simulink library "MonoizerLib"  (R2022b)
settings: Solver=VariableStepAuto  StartTime=0.0  StopTime=10.0  RelTol=1e-3
libraries: TuneVar x2, dspindex x2, HandyTextFile x1, matrix_library x1
settings Model: Creator=jb1046154  LastModifiedBy=sa1045272
settings SolverCC: AlgebraicLoopSolver=TrustRegion
settings DebuggingCC: UnconnectedInputMsg=warning  UnconnectedOutputMsg=warning  UnconnectedLineMsg=warning  SFMachineParentedDataDiag=warning
settings ModelReferenceCC: EnableRefExpFcnMdlSchedulingChecks=on

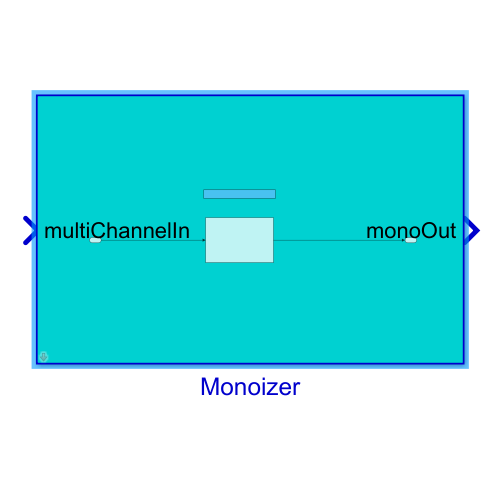
[thumbnail: Simulink's stored preview of the top-level diagram]
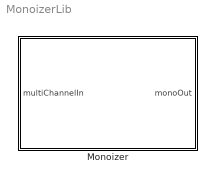
== system MonoizerLib ==
  Monoizer : Subsystem  mask(Monoizer){Config=[]}
      mask prompts: Config "MonoizerConfig"
      mask help:
      | This mask allows the setting of parameters for the Monoizer model.
      | Model parameters are set by a class instance in the base workspace.
      |
      | See 'Help' for details.
      mask init:
      | blkh=gcbh;
      | Config=BTConfig.Assert(blkh,Config);
      | 
      | Config.Validate();
      | Config.DoMaskInit(blkh);
      mask Help:
      | Defining model parameters:
      | The model parameters are set by the conents of an instance of MonoizerClass.m.
      | 
      | To set model parameters:
      | 1-Create an instance of MonoizerClass.m in the base workspace.
      | 2-In the model mask, set the 'Class instance' parameter to the name of the class instance in the base workspace.

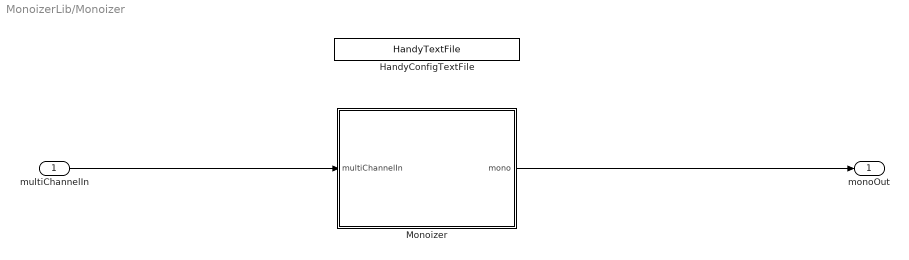
== system MonoizerLib/Monoizer ==
  multiChannelIn : Inport
  HandyConfigTextFile : HandyTextFile/HandyTextFile  TemplateSource=Config  FileSuffix=File  OpenDialogOnLoad=off  UseThisBlockName=off  AddGrandParentNamePrefix=off  TheDefaultText=% $(FILENAME) $(PREFIX) $(SUFFIX)  ShowInLibBrowser=on
      settings: SourceProductName=Bose Talaria
  Monoizer : Subsystem  Variant=on  VariantControl=Choice
  monoOut : Outport  VectorParamsAs1DForOutWhenUnconnected=off
  wires:
  multiChannelIn/1 -> Monoizer/1(multiChannelIn)
  Monoizer/1(mono) -> monoOut/1

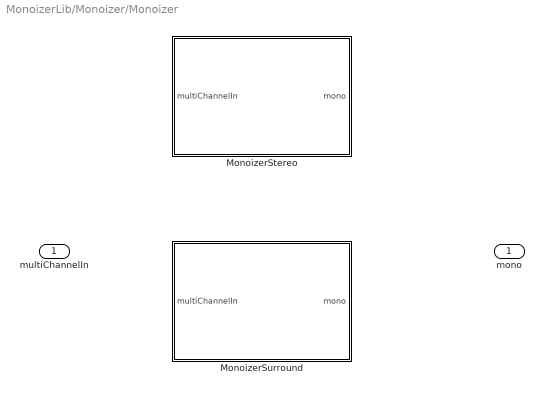
== system MonoizerLib/Monoizer/Monoizer ==
  multiChannelIn : Inport
  MonoizerStereo : Subsystem  VariantControl=Config.NumChannels == 2
  MonoizerSurround : Subsystem  VariantControl=Config.NumChannels > 2
  mono : Outport

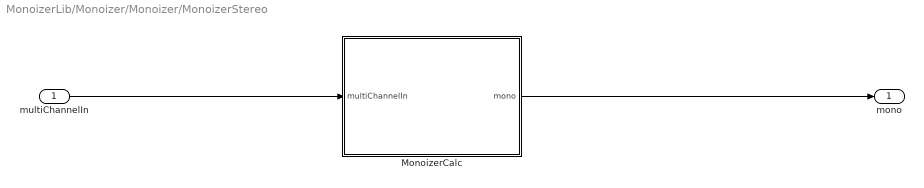
== system MonoizerLib/Monoizer/Monoizer/MonoizerStereo ==
  multiChannelIn : Inport
  MonoizerCalc : Subsystem
  mono : Outport
  wires:
  multiChannelIn/1 -> MonoizerCalc/1(multiChannelIn)
  MonoizerCalc/1(mono) -> mono/1

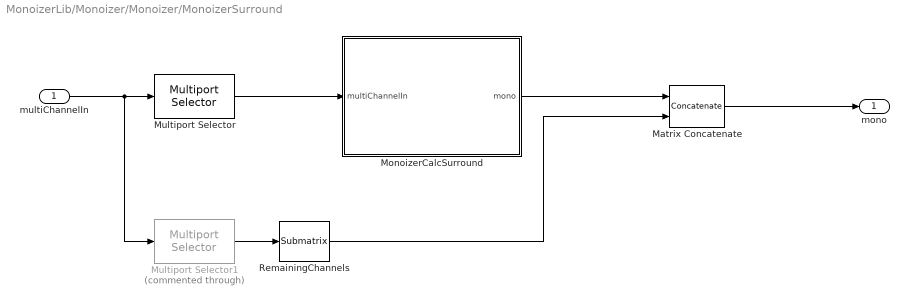
== system MonoizerLib/Monoizer/Monoizer/MonoizerSurround ==
  multiChannelIn : Inport
  Matrix Concatenate : Concatenate  Mode=Multidimensional array  ConcatenateDimension=2
  MonoizerCalcSurround : Subsystem
  Multiport Selector : dspindex/Multiport Selector  rowsOrCols=Columns  idxCellArray={1:2}  idxErrMode=Clip Index
      settings: LibrarySourceBlock=|
      | dsphdlsupportsigmgmt/Multiport
      | Selector
  Multiport Selector1 : dspindex/Multiport Selector  Commented=through  rowsOrCols=Columns  idxCellArray=3:4  idxErrMode=Clip and Warn
      settings: LibrarySourceBlock=|
      | dsphdlsupportsigmgmt/Multiport
      | Selector
  RemainingChannels : matrix_library/Submatrix  RowSpan=All rows  RowStartMode=First  RowStartIndex=1  RowEndMode=Last  RowEndIndex=1  ColSpan=Range of columns  ColStartMode=Index  ColStartIndex=3  ColEndMode=Last  ColEndIndex=1
  mono : Outport
  wires:
  multiChannelIn/1 -> Multiport Selector1/1, Multiport Selector/1
  MonoizerCalcSurround/1(mono) -> Matrix Concatenate/1
  Multiport Selector/1 -> MonoizerCalcSurround/1(multiChannelIn)
  Matrix Concatenate/1 -> mono/1
  RemainingChannels/1 -> Matrix Concatenate/2
  Multiport Selector1/1 -> RemainingChannels/1

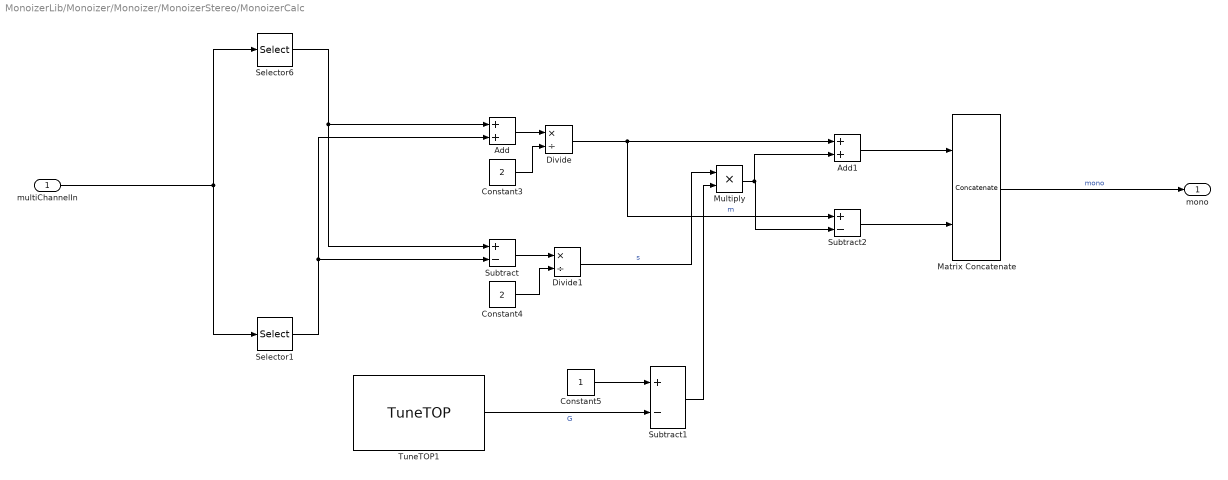
== system MonoizerLib/Monoizer/Monoizer/MonoizerStereo/MonoizerCalc ==
  multiChannelIn : Inport
  Add : Sum
  Add1 : Sum
  Constant3 : Constant  Value=2  OutDataTypeStr=single
  Constant4 : Constant  Value=2  OutDataTypeStr=single
  Constant5 : Constant  OutDataTypeStr=single
  Divide : Product  Inputs=*/  RndMeth=Zero  SaturateOnIntegerOverflow=on
  Divide1 : Product  Inputs=*/  RndMeth=Zero  SaturateOnIntegerOverflow=on
  Matrix Concatenate : Concatenate  Mode=Multidimensional array  ConcatenateDimension=2
  Multiply : Product
  Selector1 : Selector  NumberOfDimensions=2  InputPortWidth=3  IndexOptions=Select all,Index vector (dialog)  Indices=4,2  OutputSizes=1,1
  Selector6 : Selector  NumberOfDimensions=2  InputPortWidth=3  IndexOptions=Select all,Index vector (dialog)  Indices=4,1  OutputSizes=1,1
  Subtract : Sum  Inputs=+-
  Subtract1 : Sum  Inputs=+-
  Subtract2 : Sum  Inputs=+-
  TuneTOP1 : TuneVar/TuneTOP  TriggerInit=[385 412 535 498]  TopName=G  TuneName=G  DataType=single  TunabilityNumber=1  MinValue=[]  MaxValue=[]  BankNumber=0  PreOverlay=false  PostOverlay=false  UseSameName=on  MaskValue=Config.G
      settings: SourceProductName=Bose Talaria
  mono : Outport
  wires:
  multiChannelIn/1 -> Selector6/1, Selector1/1
  Subtract1/1 -> Multiply/2
  Constant4/1 -> Divide1/2
  Selector6/1 -> Subtract/1, Add/1
  Add1/1 -> Matrix Concatenate/1
  TuneTOP1/1 -> Subtract1/2  "G"
  Subtract/1 -> Divide1/1
  Divide/1 -> Subtract2/1, Add1/1  "m"
  Constant5/1 -> Subtract1/1
  Constant3/1 -> Divide/2
  Subtract2/1 -> Matrix Concatenate/2
  Add/1 -> Divide/1
  Matrix Concatenate/1 -> mono/1  "mono"
  Multiply/1 -> Subtract2/2, Add1/2
  Divide1/1 -> Multiply/1  "s"
  Selector1/1 -> Add/2, Subtract/2

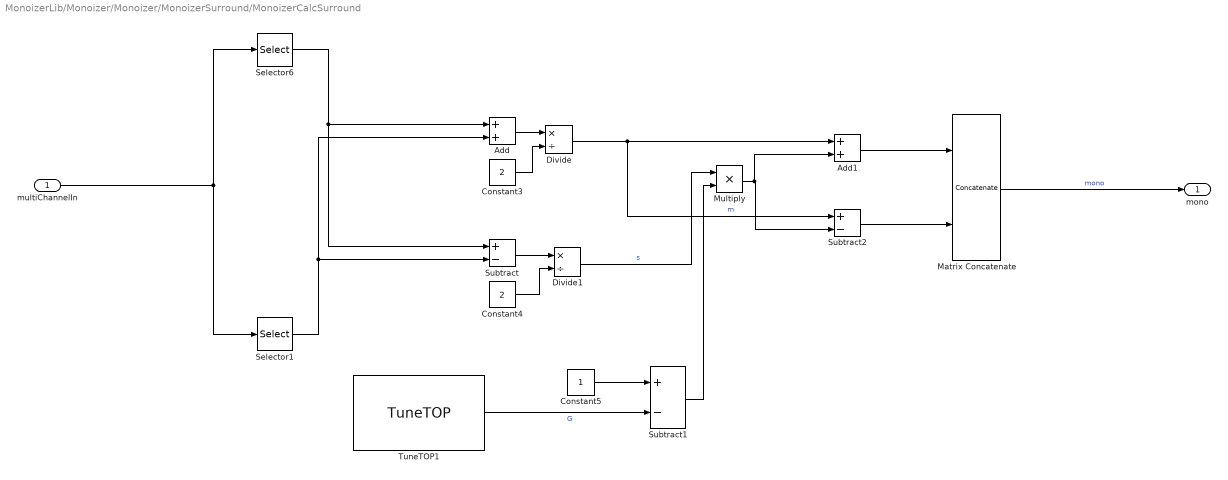
== system MonoizerLib/Monoizer/Monoizer/MonoizerSurround/MonoizerCalcSurround ==
  multiChannelIn : Inport
  Add : Sum
  Add1 : Sum
  Constant3 : Constant  Value=2  OutDataTypeStr=single
  Constant4 : Constant  Value=2  OutDataTypeStr=single
  Constant5 : Constant  OutDataTypeStr=single
  Divide : Product  Inputs=*/  RndMeth=Zero  SaturateOnIntegerOverflow=on
  Divide1 : Product  Inputs=*/  RndMeth=Zero  SaturateOnIntegerOverflow=on
  Matrix Concatenate : Concatenate  Mode=Multidimensional array  ConcatenateDimension=2
  Multiply : Product
  Selector1 : Selector  NumberOfDimensions=2  InputPortWidth=3  IndexOptions=Select all,Index vector (dialog)  Indices=4,2  OutputSizes=1,1
  Selector6 : Selector  NumberOfDimensions=2  InputPortWidth=3  IndexOptions=Select all,Index vector (dialog)  Indices=4,1  OutputSizes=1,1
  Subtract : Sum  Inputs=+-
  Subtract1 : Sum  Inputs=+-
  Subtract2 : Sum  Inputs=+-
  TuneTOP1 : TuneVar/TuneTOP  TriggerInit=[685 537 835 623]  TopName=G  TuneName=G  DataType=single  TunabilityNumber=1  MinValue=[]  MaxValue=[]  BankNumber=0  PreOverlay=false  PostOverlay=false  UseSameName=on  MaskValue=Config.G
      settings: SourceProductName=Bose Talaria
  mono : Outport
  wires:
  multiChannelIn/1 -> Selector6/1, Selector1/1
  Subtract1/1 -> Multiply/2
  Constant4/1 -> Divide1/2
  Selector6/1 -> Subtract/1, Add/1
  Add1/1 -> Matrix Concatenate/1
  TuneTOP1/1 -> Subtract1/2  "G"
  Subtract/1 -> Divide1/1
  Divide/1 -> Subtract2/1, Add1/1  "m"
  Constant5/1 -> Subtract1/1
  Constant3/1 -> Divide/2
  Subtract2/1 -> Matrix Concatenate/2
  Add/1 -> Divide/1
  Matrix Concatenate/1 -> mono/1  "mono"
  Multiply/1 -> Subtract2/2, Add1/2
  Divide1/1 -> Multiply/1  "s"
  Selector1/1 -> Add/2, Subtract/2
